simulink model "IM_GFLI_CC_5kW"  (R2024b)
settings: Solver=ode4  StartTime=0.0  StopTime=5  FixedStep=50e-6  RelTol=1e-3
values from neighbouring files (symbols this model uses):
  Avsc = Ast + Bst*R3*inv(eye(6) - Dst*R3)*Cst    [CCM_based_Impedance.m]    (also in CC_PLL_GFLI.m = Ast + Bst*R_3*inv(eye(6) - Dst*R_3)*Cst; CC_PLL_GFLI_Plot.m = Ast + Bst*R_3*inv(eye(6) - Dst*R_3)*Cst)
  Bvsc = Bst*R3*inv(eye(6)-Dst*R3)*Dst*R2 + Bst*R2    [CCM_based_Impedance.m]    (also in CC_PLL_GFLI.m = Bst*R_3*inv(eye(6)-Dst*R_3)*Dst*R_2 + Bst*R_2; CC_PLL_GFLI_Plot.m = Bst*R_3*inv(eye(6)-Dst*R_3)*Dst*R_2 + Bst*R_2)
  Cf = 50e-6    (= 5e-05)    [CCM_based_Impedance.m]    (also in CC_PLL_GFLI.m; CC_PLL_GFLI_Plot.m)
  Cvsc = R1*inv(eye(6)-Dst*R3)*Cst    [CCM_based_Impedance.m]    (also in CC_PLL_GFLI.m = R_1*inv(eye(6)-Dst*R_3)*Cst; CC_PLL_GFLI_Plot.m = R_1*inv(eye(6)-Dst*R_3)*Cst)
  Dvsc = R1*inv(eye(6)-Dst*R3)*Dst*R2+R0    [CCM_based_Impedance.m]    (also in CC_PLL_GFLI.m = R_1*inv(eye(6)-Dst*R_3)*Dst*R_2+R_0; CC_PLL_GFLI_Plot.m = R_1*inv(eye(6)-Dst*R_3)*Dst*R_2+R_0)
  Kii = 0.0348    [CCM_based_Impedance.m]    (also in CC_PLL_GFLI.m; CC_PLL_GFLI_Plot.m)
  Kipll = 200    [CCM_based_Impedance.m]    (also in CC_PLL_GFLI.m = 0.347826086957; CC_PLL_GFLI_Plot.m = 0.347826086957)
  Kpi = 1.7391e-4    (= 0.00017391)    [CCM_based_Impedance.m]    (also in CC_PLL_GFLI.m; CC_PLL_GFLI_Plot.m)
  Kppll = 20    [CCM_based_Impedance.m]    (also in CC_PLL_GFLI.m = 0.0347826086957; CC_PLL_GFLI_Plot.m = 0.0347826086957)
  Lf1 = 250e-6    (= 0.00025)    [CCM_based_Impedance.m]    (also in CC_PLL_GFLI.m; CC_PLL_GFLI_Plot.m)
  Lf2 = 250e-6    (= 0.00025)    [CCM_based_Impedance.m]    (also in CC_PLL_GFLI.m; CC_PLL_GFLI_Plot.m)
  Rf1 = 3e-3    (= 0.003)    [CCM_based_Impedance.m]    (also in CC_PLL_GFLI.m; CC_PLL_GFLI_Plot.m)
  Rf2 = 3e-3    (= 0.003)    [CCM_based_Impedance.m]    (also in CC_PLL_GFLI.m; CC_PLL_GFLI_Plot.m)
  Td = 1.5*Ts    (= 0.0003)    [CCM_based_Impedance.m]    (also in CC_PLL_GFLI.m; CC_PLL_GFLI_Plot.m)
  Vdc = 1150    [CCM_based_Impedance.m]    (also in CC_PLL_GFLI.m; CC_PLL_GFLI_Plot.m)
  w1 = 100*pi    (= 314.159265359)    [CCM_based_Impedance.m]    (also in CC_PLL_GFLI.m; CC_PLL_GFLI_Plot.m)
libraries: spsSeriesRLCBranchLib x12, spsVoltageMeasurementLib x6, spsACVoltageSourceLib x3, spsControlledVoltageSourceLib x3, spsCurrentMeasurementLib x3, spsabctodq0Lib x2, spsGroundLib x1, spsdq0toabcLib x1, sps_lib x1
settings Model: Creator=ACER  LastModifiedBy=ACER
settings DataIOCC: SaveFormat=StructureWithTime  SignalLogging=off  DSMLogging=off  SaveTime=off  ReturnWorkspaceOutputs=off

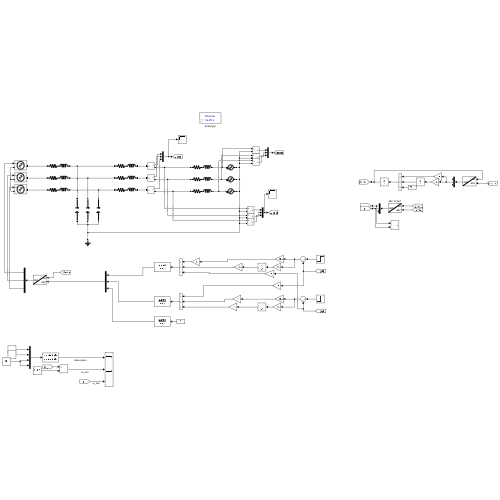
[thumbnail: Simulink's stored preview of the top-level diagram]
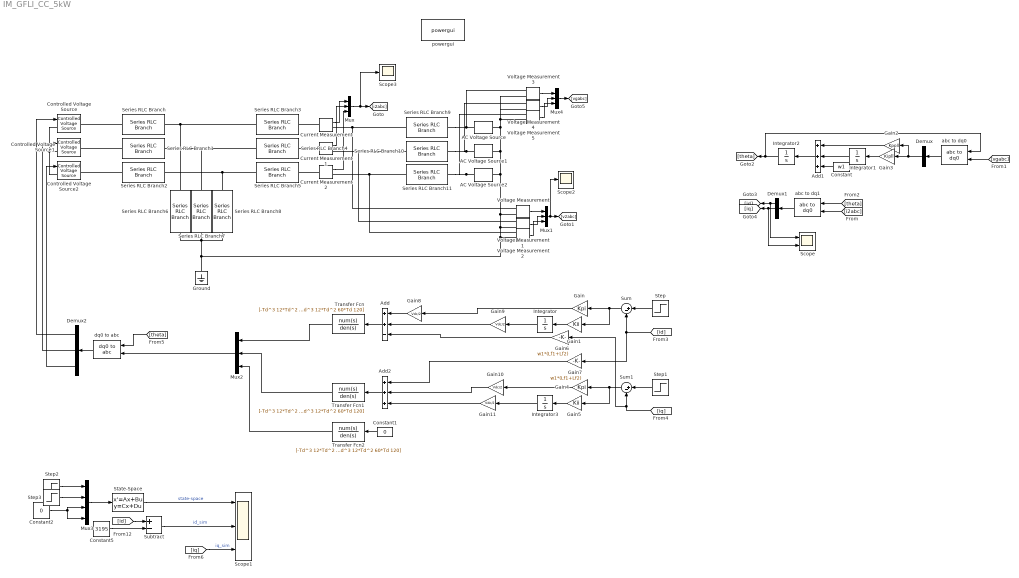
== system IM_GFLI_CC_5kW ==
  AC Voltage Source : spsACVoltageSourceLib/AC Voltage Source  Amplitude=575  Phase=0  Frequency=50  SampleTime=0  Measurements=None  BusType=swing  Pref=10e3  Qref=0  Qmin=-inf  Qmax=+inf
  AC Voltage Source1 : spsACVoltageSourceLib/AC Voltage Source  Amplitude=575  Phase=-120  Frequency=50  SampleTime=0  Measurements=None  BusType=swing  Pref=10e3  Qref=0  Qmin=-inf  Qmax=+inf
  AC Voltage Source2 : spsACVoltageSourceLib/AC Voltage Source  Amplitude=575  Phase=120  Frequency=50  SampleTime=0  Measurements=None  BusType=swing  Pref=10e3  Qref=0  Qmin=-inf  Qmax=+inf
  Add : Sum  Inputs=++-
  Add1 : Sum  Inputs=+++
  Add2 : Sum  Inputs=+++
  Constant : Constant  Value=w1
  Constant1 : Constant  Value=0
  Constant2 : Constant  Value=0
  Constant5 : Constant  Value=3195
  Controlled Voltage Source : spsControlledVoltageSourceLib/Controlled Voltage Source  Initialize=on  Source_Type=AC  Amplitude=0  Phase=0  Frequency=0  Measurements=None
  Controlled Voltage Source1 : spsControlledVoltageSourceLib/Controlled Voltage Source  Initialize=on  Source_Type=AC  Amplitude=0  Phase=0  Frequency=0  Measurements=None
  Controlled Voltage Source2 : spsControlledVoltageSourceLib/Controlled Voltage Source  Initialize=on  Source_Type=AC  Amplitude=0  Phase=0  Frequency=0  Measurements=None
  Current Measurement : spsCurrentMeasurementLib/Current Measurement  PhasorSimulation=off  OutputType=Complex  PSBequivalent=0
  Current Measurement1 : spsCurrentMeasurementLib/Current Measurement  PhasorSimulation=off  OutputType=Complex  PSBequivalent=0
  Current Measurement2 : spsCurrentMeasurementLib/Current Measurement  PhasorSimulation=off  OutputType=Complex  PSBequivalent=0
  Demux : Demux  Outputs=3
  Demux1 : Demux  Outputs=3
  Demux2 : Demux  Outputs=3
  Gain : Gain  Gain=Kpi
  Gain1 : Gain  Gain=Kii
  Gain{8..11} (4 alike) : Gain  Gain=Vdc/2
  Gain2 : Gain  Gain=Kppll
  Gain3 : Gain  Gain=Kipll
  Gain4 : Gain  Gain=Kpi
  Gain5 : Gain  Gain=Kii
  Gain6 : Gain  Gain=w1*(Lf1+Lf2)
  Gain7 : Gain  Gain=w1*(Lf1+Lf2)
  Ground : spsGroundLib/Ground  LConnTagsString=a
  Integrator{,1..3} (4 alike) : Integrator
  Mux{,1..2,4} (4 alike) : Mux  Inputs=3
  Mux3 : Mux
  Scope : Scope  NumInputPorts=2
  Scope1 : Scope  NumInputPorts=3
  Scope2 : Scope
  Scope3 : Scope
  Series RLC Branch : spsSeriesRLCBranchLib/Series RLC Branch  LConnTagsString=__new0  RConnTagsString=__new0  BranchType=RL  Resistance=Rf1  Inductance=Lf1  SetiL0=off  InitialCurrent=0  Capacitance=1e-6  Setx0=off  InitialVoltage=0  Measurements=None
  Series RLC Branch1 : spsSeriesRLCBranchLib/Series RLC Branch  LConnTagsString=__new0  RConnTagsString=__new0  BranchType=RL  Resistance=Rf1  Inductance=Lf1  SetiL0=off  InitialCurrent=0  Capacitance=1e-6  Setx0=off  InitialVoltage=0  Measurements=None
  Series RLC Branch10 : spsSeriesRLCBranchLib/Series RLC Branch  LConnTagsString=__new0  RConnTagsString=__new0  BranchType=RL  Resistance=Rf2  Inductance=Lf2*20  SetiL0=off  InitialCurrent=0  Capacitance=1e-6  Setx0=off  InitialVoltage=0  Measurements=None
  Series RLC Branch11 : spsSeriesRLCBranchLib/Series RLC Branch  LConnTagsString=__new0  RConnTagsString=__new0  BranchType=RL  Resistance=Rf2  Inductance=Lf2*20  SetiL0=off  InitialCurrent=0  Capacitance=1e-6  Setx0=off  InitialVoltage=0  Measurements=None
  Series RLC Branch2 : spsSeriesRLCBranchLib/Series RLC Branch  LConnTagsString=__new0  RConnTagsString=__new0  BranchType=RL  Resistance=Rf1  Inductance=Lf1  SetiL0=off  InitialCurrent=0  Capacitance=1e-6  Setx0=off  InitialVoltage=0  Measurements=None
  Series RLC Branch3 : spsSeriesRLCBranchLib/Series RLC Branch  LConnTagsString=__new0  RConnTagsString=__new0  BranchType=RL  Resistance=Rf2  Inductance=Lf2  SetiL0=off  InitialCurrent=0  Capacitance=1e-6  Setx0=off  InitialVoltage=0  Measurements=None
  Series RLC Branch4 : spsSeriesRLCBranchLib/Series RLC Branch  LConnTagsString=__new0  RConnTagsString=__new0  BranchType=RL  Resistance=Rf2  Inductance=Lf2  SetiL0=off  InitialCurrent=0  Capacitance=1e-6  Setx0=off  InitialVoltage=0  Measurements=None
  Series RLC Branch5 : spsSeriesRLCBranchLib/Series RLC Branch  LConnTagsString=__new0  RConnTagsString=__new0  BranchType=RL  Resistance=Rf2  Inductance=Lf2  SetiL0=off  InitialCurrent=0  Capacitance=1e-6  Setx0=off  InitialVoltage=0  Measurements=None
  Series RLC Branch6 : spsSeriesRLCBranchLib/Series RLC Branch  LConnTagsString=__new0  RConnTagsString=__new0  BranchType=C  Resistance=Rf2  Inductance=Lf2  SetiL0=off  InitialCurrent=0  Capacitance=Cf  Setx0=off  InitialVoltage=0  Measurements=None
  Series RLC Branch7 : spsSeriesRLCBranchLib/Series RLC Branch  LConnTagsString=__new0  RConnTagsString=__new0  BranchType=C  Resistance=Rf2  Inductance=Lf2  SetiL0=off  InitialCurrent=0  Capacitance=Cf  Setx0=off  InitialVoltage=0  Measurements=None
  Series RLC Branch8 : spsSeriesRLCBranchLib/Series RLC Branch  LConnTagsString=__new0  RConnTagsString=__new0  BranchType=C  Resistance=Rf2  Inductance=Lf2  SetiL0=off  InitialCurrent=0  Capacitance=Cf  Setx0=off  InitialVoltage=0  Measurements=None
  Series RLC Branch9 : spsSeriesRLCBranchLib/Series RLC Branch  LConnTagsString=__new0  RConnTagsString=__new0  BranchType=RL  Resistance=Rf2  Inductance=Lf2*20  SetiL0=off  InitialCurrent=0  Capacitance=1e-6  Setx0=off  InitialVoltage=0  Measurements=None
  State-Space : StateSpace  A=Avsc  B=Bvsc  C=Cvsc  D=Dvsc  InitialCondition=0
  Step : Step  Time=2  Before=3195  After=3408  SampleTime=0
  Step1 : Step  Time=3  After=426  SampleTime=0
  Step2 : Step  Time=2  After=213  SampleTime=0
  Step3 : Step  Time=3  After=426  SampleTime=0
  Subtract : Sum  Inputs=+-
  Sum : Sum  Inputs=|+-
  Sum1 : Sum  Inputs=|+-
  Transfer Fcn : TransferFcn  Numerator=[-Td^3 12*Td^2 -60*Td 120]  Denominator=[Td^3 12*Td^2 60*Td 120]
  Transfer Fcn1 : TransferFcn  Numerator=[-Td^3 12*Td^2 -60*Td 120]  Denominator=[Td^3 12*Td^2 60*Td 120]
  Transfer Fcn2 : TransferFcn  Numerator=[-Td^3 12*Td^2 -60*Td 120]  Denominator=[Td^3 12*Td^2 60*Td 120]
  Voltage Measurement{,1..5} (6 alike) : spsVoltageMeasurementLib/Voltage Measurement  PhasorSimulation=off  OutputType=Complex  PSBequivalent=0
  abc to dq0 : spsabctodq0Lib/abc to dq0  Alignment=Aligned with phase A axis
  abc to dq1 : spsabctodq0Lib/abc to dq0  Alignment=Aligned with phase A axis
  dq0 to abc : spsdq0toabcLib/dq0 to abc  Alignment=Aligned with phase A axis
  powergui : sps_lib/powergui  Priority=1  SimulationMode=Discrete  SampleTime=50e-6  frequency=60  Iterations=50  frequencyindice=50  Pbase=100e6  ErrMax=1e-4  UnitsV=kV  UnitsW=MW  buscounter=0  FunctionMessages=off  echomessages=off  EnableUseOfTLC=off  CurrentSourceSwitches=off  DisableSnubberDevices=off  DisableRonSwitches=off  DisableVfSwitches=off  DisplayEquations=off  AutomaticDiscreteSolvers=off  SolverType=Tustin/Backward Euler (TBE)  Interpol=off  ExternalGateDelay=off  methode=off  Ts=100  x0status=blocks  SPID=on  SwTol=0  HookPort=off  NonlinearTolerance=1e-4  nMaxIteration=100  ContinueOnMaxIteration=off  RestoreLinks=warning  ResistiveCurrentMeasurement=off  Frange=[0:2:500]  Ylog=off  Xlog=on  ShowGrid=off  save=off  variable=ZData  structure=0  ZoomFFT=off  StartTime=0.0  cycles=1  DisplayStyle=1  fundamental=60  FreqAxis=off  MaxFrequency=1000  frequencyindicesteady=1  RmsSteady=1  display=off
  wires:
  Sum/1 -> Gain1/1, Gain/1
  Gain1/1 -> Integrator/1
  Gain/1 -> Gain8/1
  Integrator/1 -> Gain9/1
  Step/1 -> Sum/1
  Current Measurement/1 -> Mux/1
  Current Measurement1/1 -> Mux/2
  Current Measurement2/1 -> Mux/3
  Mux/1 -> Scope3/1, [i2abc]
  Voltage Measurement/1 -> Mux1/1
  Voltage Measurement1/1 -> Mux1/2
  Voltage Measurement2/1 -> Mux1/3
  Mux1/1 -> Scope2/1, [v2abc]
  [vgabc] -> abc to dq0/1
  abc to dq0/1 -> Demux/1
  Gain2/1 -> Add1/1
  Gain3/1 -> Integrator1/1
  Demux/2 -> Gain2/1, Gain3/1
  Integrator1/1 -> Add1/2
  Constant/1 -> Add1/3
  Add1/1 -> Integrator2/1
  Integrator2/1 -> abc to dq0/2, [theta]
  [i2abc] -> abc to dq1/1
  [theta] -> abc to dq1/2
  abc to dq1/1 -> Demux1/1
  Demux1/1 -> Scope/1, [id]
  Demux1/2 -> Scope/2, [iq]
  [id] -> Sum/2, Gain7/1
  [iq] -> Gain6/1, Sum1/2
  Step1/1 -> Sum1/1
  Gain5/1 -> Integrator3/1
  Sum1/1 -> Gain4/1, Gain5/1
  Integrator3/1 -> Gain11/1
  Gain4/1 -> Gain10/1
  Constant1/1 -> Transfer Fcn2/1
  dq0 to abc/1 -> Demux2/1
  Demux2/1 -> Controlled Voltage Source/1
  Demux2/2 -> Controlled Voltage Source1/1
  Demux2/3 -> Controlled Voltage Source2/1
  [theta] -> dq0 to abc/2
  Mux3/1 -> State-Space/1
  Step2/1 -> Mux3/1
  Step3/1 -> Mux3/2
  Constant2/1 -> Mux3/4, Mux3/3
  State-Space/1 -> Scope1/1  "state-space"
  [id] -> Subtract/1
  Constant5/1 -> Subtract/2
  Subtract/1 -> Scope1/2  "id_sim"
  Gain6/1 -> Add/3
  Gain7/1 -> Add2/1
  Add/1 -> Transfer Fcn/1
  Add2/1 -> Transfer Fcn1/1
  Mux2/1 -> dq0 to abc/1
  Transfer Fcn/1 -> Mux2/1
  Transfer Fcn1/1 -> Mux2/2
  Transfer Fcn2/1 -> Mux2/3
  Gain8/1 -> Add/1
  Gain9/1 -> Add/2
  Gain10/1 -> Add2/2
  Gain11/1 -> Add2/3
  [iq] -> Scope1/3  "iq_sim"
  Mux4/1 -> [vgabc]
  Voltage Measurement5/1 -> Mux4/3
  Voltage Measurement4/1 -> Mux4/2
  Voltage Measurement3/1 -> Mux4/1
  connections:
  Controlled Voltage Source/LConn1 -- Controlled Voltage Source1/LConn1 -- Controlled Voltage Source2/LConn1
  Series RLC Branch/LConn1 -- Controlled Voltage Source/RConn1
  Series RLC Branch1/LConn1 -- Controlled Voltage Source1/RConn1
  Series RLC Branch2/LConn1 -- Controlled Voltage Source2/RConn1
  Series RLC Branch3/LConn1 -- Series RLC Branch6/LConn1 -- Series RLC Branch/RConn1
  Series RLC Branch4/LConn1 -- Series RLC Branch7/LConn1 -- Series RLC Branch1/RConn1
  Series RLC Branch5/LConn1 -- Series RLC Branch8/LConn1 -- Series RLC Branch2/RConn1
  AC Voltage Source/LConn1 -- Voltage Measurement3/LConn2 -- Voltage Measurement4/LConn2 -- Voltage Measurement5/LConn2 -- AC Voltage Source1/LConn1 -- AC Voltage Source2/LConn1 -- Voltage Measurement1/LConn2 -- Voltage Measurement2/LConn2 -- Series RLC Branch7/RConn1 -- Series RLC Branch6/RConn1 -- Series RLC Branch8/RConn1 -- Ground/LConn1 -- Voltage Measurement/LConn2
  Current Measurement/LConn1 -- Series RLC Branch3/RConn1
  Voltage Measurement/LConn1 -- Series RLC Branch9/LConn1 -- Current Measurement/RConn1
  Current Measurement1/LConn1 -- Series RLC Branch4/RConn1
  Current Measurement2/LConn1 -- Series RLC Branch5/RConn1
  Voltage Measurement1/LConn1 -- Series RLC Branch10/LConn1 -- Current Measurement1/RConn1
  Voltage Measurement2/LConn1 -- Series RLC Branch11/LConn1 -- Current Measurement2/RConn1
  Series RLC Branch9/RConn1 -- Voltage Measurement3/LConn1 -- AC Voltage Source/RConn1
  AC Voltage Source1/RConn1 -- Series RLC Branch10/RConn1 -- Voltage Measurement4/LConn1
  AC Voltage Source2/RConn1 -- Series RLC Branch11/RConn1 -- Voltage Measurement5/LConn1
